simulink model "PMDC"  (R2020b)
settings: Solver=VariableStepAuto  StartTime=0.0  StopTime=10.0  RelTol=1e-3
undefined symbols (not defined in the file): b, J, K, L, R
settings Model: Creator=orangejuzi  LastModifiedBy=orangejuzi

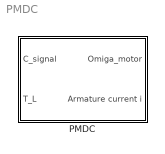
== system PMDC ==
  PMDC : Subsystem

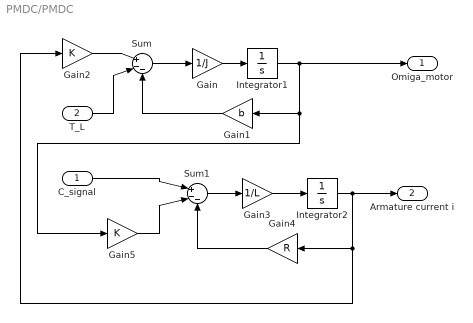
== system PMDC/PMDC ==
  C_signal : Inport
  T_L : Inport  Port=2
  Gain : Gain  Gain=1/J
  Gain1 : Gain  Gain=b
  Gain2 : Gain  Gain=K
  Gain3 : Gain  Gain=1/L
  Gain4 : Gain  Gain=R
  Gain5 : Gain  Gain=K
  Integrator1 : Integrator
  Integrator2 : Integrator
  Sum : Sum  Inputs=|+--
  Sum1 : Sum  Inputs=|+--
  Omiga_motor : Outport
  Armature current i : Outport  Port=2
  wires:
  Sum/1 -> Gain/1
  Gain/1 -> Integrator1/1
  Gain1/1 -> Sum/3
  T_L/1 -> Sum/2
  Integrator2/1 -> Gain4/1, Gain2/1, Armature current i/1
  Gain2/1 -> Sum/1
  Sum1/1 -> Gain3/1
  Gain3/1 -> Integrator2/1
  C_signal/1 -> Sum1/1
  Integrator1/1 -> Omiga_motor/1, Gain1/1, Gain5/1
  Gain4/1 -> Sum1/3
  Gain5/1 -> Sum1/2
